simulink model "caoxing_MPC_demo"  (R2020a)
settings: Solver=FixedStepDiscrete  StartTime=0.0  StopTime=10  FixedStep=0.01  RelTol=1e-3  EnableMultiTasking=on
PostLoadFcn:
  | K1 = 2; K2 = int8(3); MYTYPE = Simulink.AliasType('single');
Description:
  | Context-Sensitive Parameters in C-MEX S-functions
settings Model: ExtModeAutoUpdateStatusClock=off  TunableVars=K1,K2  TunableVarsStorageClass=ExportedGlobal,ExportedGlobal  TunableVarsTypeQualifier=,  Creator=The MathWorks, Inc.  LastModifiedBy=root
settings DataIOCC: LimitDataPoints=on  SaveFormat=Array  SaveOutput=off  SaveTime=off  SignalLoggingName=sigsOut
settings OptimizationCC: DefaultParameterBehavior=Inlined  ExpressionDepthLimit=2147483647  StateBitsets=on  DataBitsets=on  InitFltsAndDblsToZero=on  LifeSpan=inf  BufferReusableBoundary=off
settings DebuggingCC: SaveWithParameterizedLinksMsg=none  CheckExecutionContextPreStartOutputMsg=on  CheckExecutionContextRuntimeOutputMsg=on  MultiTaskDSMMsg=warning  MultiTaskCondExecSysMsg=none  FcnCallInpInsideContextMsg=warning  AllowSymbolicDim=off  StateNameClashWarn=warning  SFUnexpectedBacktrackingDiag=warning  SFNoUnconditionalDefaultTransitionDiag=warning  SFExecutionAtInitializationDiag=none  ArithmeticOperatorsInVariantConditions=warning
settings HardwareCC: ProdBitPerPointer=32  ProdBitPerSizeT=32  ProdBitPerPtrDiffT=32  ProdLargestAtomicFloat=None  ProdIntDivRoundTo=Undefined  ProdEndianess=Unspecified  ProdWordSize=32  ProdHWDeviceType=32-bit Generic
settings ModelReferenceCC: PropagateSignalLabelsOutOfModel=off
settings SFSimCC: SimUseLocalCustomCode=off  SimParseCustomCode=off  CustomCodeUndefinedFunction=UseInterfaceOnly
settings RTWCC: Description=Generic Real-Time Target  TLCOptions=-p0  GenerateReport=on  RTWUseLocalCustomCode=off  LaunchReport=on
settings CodeAppCC: ForceParamTrailComments=on  StateflowObjectComments=on
settings GRTTargetCC: TargetFcnLib=ansi_tfl_tmw.mat  TargetLangStandard=C89/C90 (ANSI)  CombineOutputUpdateFcns=off  GRTInterface=on
settings ConfigComp: CovMetricSettings=d  CovHtmlReporting=on  CovSaveCumulativeToWorkspaceVar=on  CovSaveSingleToWorkspaceVar=on  CovExternalEMLEnable=off

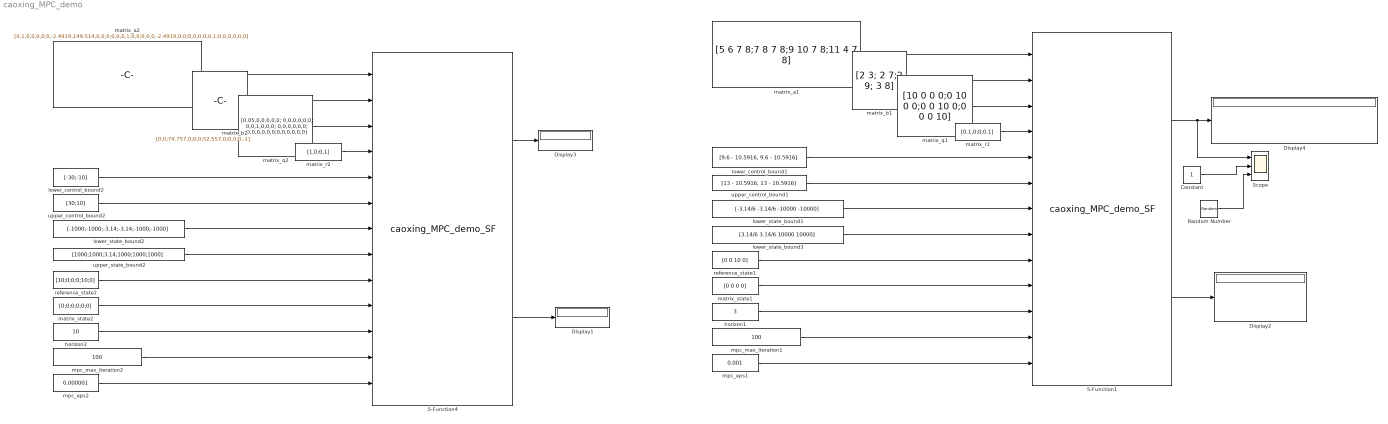
== system caoxing_MPC_demo ==
  Constant : Constant
  Display{1..4} (4 alike) : Display
      Display4 settings: Decimation=5
  Random Number : RandomNumber  SampleTime=0.1
  S-Function1 : S-Function  FunctionName=caoxing_MPC_demo_SF  Parameters=basic_state_size, controls  SFunctionDeploymentMode=off  EnableBusSupport=off  mask{basic_state_size=4, controls=2}
  S-Function4 : S-Function  FunctionName=caoxing_MPC_demo_SF  Parameters=basic_state_size, controls  SFunctionDeploymentMode=off  EnableBusSupport=off  mask{basic_state_size=6, controls=2}
  Scope : Scope  NumInputPorts=3
  horizon1 : Constant  Value=3  OutDataTypeStr=double
  horizon2 : Constant  Value=10  OutDataTypeStr=double
  lower_control_bound1 : Constant  Value=[9.6 - 10.5916, 9.6 - 10.5916]  OutDataTypeStr=double
  lower_control_bound2 : Constant  Value=[-30;-10]  OutDataTypeStr=double
  lower_state_bound1 : Constant  Value=[-3.14/6 -3.14/6 -10000 -10000]  OutDataTypeStr=double
  lower_state_bound2 : Constant  Value=[-1000;-1000;-3.14;-3.14;-1000;-1000]  OutDataTypeStr=double
  lower_state_bound3 : Constant  Value=[3.14/6 3.14/6 10000 10000]  OutDataTypeStr=double
  matrix_a1 : Constant  Value=[5 6 7 8;7 8 7 8;9 10 7 8;11 4 7 8]  OutDataTypeStr=double
  matrix_a2 : Constant  Value=[0,1,0,0,0,0;0,-2.4919,149.514,0,0,0;0,0,0,1,0,0;0,0,0,-2.4919,0,0;0,0,0,0,0,1;0,0,0,0,0,0]  OutDataTypeStr=double
  matrix_b1 : Constant  Value=[2 3; 2 7;2 9; 3 8]  OutDataTypeStr=double
  matrix_b2 : Constant  Value=[0,0;74.757,0;0,0;52.557,0;0,0;0,-1]  OutDataTypeStr=double
  matrix_q1 : Constant  Value=[10 0 0 0;0 10 0 0;0 0 10 0;0 0 0 10]  OutDataTypeStr=double
  matrix_q2 : Constant  Value="[0.05,0,0,0,0,0;  0,0,0,0,0,0;  0,0,1,0,0,0; 0,0,0,0,0,0; 0,0,0,0,0,0;0,0,0,0,0,0]"  OutDataTypeStr=double
  matrix_r1 : Constant  Value=[0.1,0;0,0.1]  OutDataTypeStr=double
  matrix_r2 : Constant  Value=[1,0;0,1]  OutDataTypeStr=double
  matrix_state1 : Constant  Value=[0 0 0 0]  OutDataTypeStr=double
  matrix_state2 : Constant  Value=[0;0;0;0;0;0]  OutDataTypeStr=double
  mpc_eps1 : Constant  Value=0.001  OutDataTypeStr=double
  mpc_eps2 : Constant  Value=0.000001  OutDataTypeStr=double
  mpc_max_iteration1 : Constant  Value=100  OutDataTypeStr=double
  mpc_max_iteration2 : Constant  Value=100  OutDataTypeStr=double
  reference_state1 : Constant  Value=[0 0 10 0]  OutDataTypeStr=double
  reference_state2 : Constant  Value=[10;0;0;0;10;0]  OutDataTypeStr=double
  upper_control_bound1 : Constant  Value=[13 - 10.5916, 13 - 10.5916]  OutDataTypeStr=double
  upper_control_bound2 : Constant  Value=[30;10]  OutDataTypeStr=double
  upper_state_bound2 : Constant  Value=[1000;1000;3.14;1000;1000;1000]  OutDataTypeStr=double
  wires:
  S-Function4/1 -> Display3/1
  matrix_a2/1 -> S-Function4/1
  matrix_b2/1 -> S-Function4/2
  matrix_r2/1 -> S-Function4/4
  matrix_q2/1 -> S-Function4/3
  lower_control_bound2/1 -> S-Function4/5
  upper_control_bound2/1 -> S-Function4/6
  lower_state_bound2/1 -> S-Function4/7
  upper_state_bound2/1 -> S-Function4/8
  reference_state2/1 -> S-Function4/9
  matrix_state2/1 -> S-Function4/10
  horizon2/1 -> S-Function4/11
  mpc_max_iteration2/1 -> S-Function4/12
  mpc_eps2/1 -> S-Function4/13
  S-Function4/2 -> Display1/1
  S-Function1/2 -> Display2/1
  mpc_eps1/1 -> S-Function1/13
  mpc_max_iteration1/1 -> S-Function1/12
  horizon1/1 -> S-Function1/11
  matrix_state1/1 -> S-Function1/10
  reference_state1/1 -> S-Function1/9
  lower_state_bound3/1 -> S-Function1/8
  lower_state_bound1/1 -> S-Function1/7
  upper_control_bound1/1 -> S-Function1/6
  lower_control_bound1/1 -> S-Function1/5
  matrix_q1/1 -> S-Function1/3
  matrix_r1/1 -> S-Function1/4
  matrix_b1/1 -> S-Function1/2
  matrix_a1/1 -> S-Function1/1
  S-Function1/1 -> Scope/1, Display4/1
  Constant/1 -> Scope/2
  Random Number/1 -> Scope/3
